simulink model "karol_kanoniczny"  (R2021b)
settings: Solver=VariableStepAuto  StartTime=0.0  StopTime=10.0  RelTol=1e-3
settings Model: Creator=radek  LastModifiedBy=radek

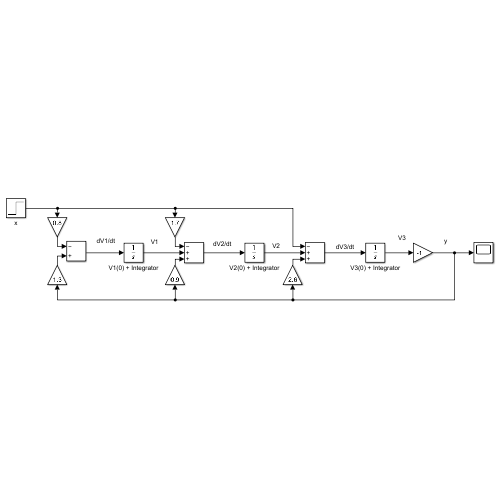
[thumbnail: Simulink's stored preview of the top-level diagram]
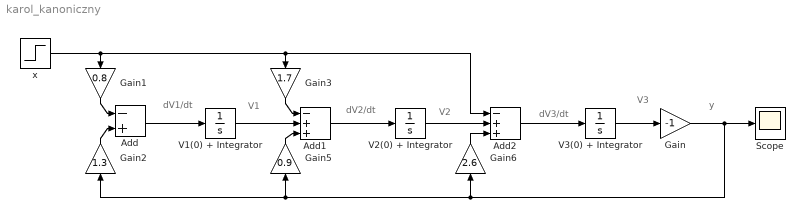
== system karol_kanoniczny ==
  note: y
  note: V3
  note: dV3/dt
  note: V2
  note: dV2/dt
  note: V1
  note: dV1/dt
  Add : Sum  Inputs=-+
  Add1 : Sum  Inputs=-++
  Add2 : Sum  Inputs=-++
  Gain : Gain  Gain=-1
  Gain1 : Gain  Gain=0.8
  Gain2 : Gain  Gain=1.3
  Gain3 : Gain  Gain=1.7
  Gain5 : Gain  Gain=0.9
  Gain6 : Gain  Gain=2.6
  Scope : Scope
  V1(0) + Integrator : Integrator
  V2(0) + Integrator : Integrator
  V3(0) + Integrator : Integrator
  x : Step  SampleTime=0
  wires:
  Gain1/1 -> Add/1
  Gain2/1 -> Add/2
  Add/1 -> V1(0) + Integrator/1
  V1(0) + Integrator/1 -> Add1/2
  Gain3/1 -> Add1/1
  Add1/1 -> V2(0) + Integrator/1
  V2(0) + Integrator/1 -> Add2/2
  x/1 -> Add2/1, Gain3/1, Gain1/1
  Add2/1 -> V3(0) + Integrator/1
  V3(0) + Integrator/1 -> Gain/1
  Gain/1 -> Gain6/1, Gain2/1, Gain5/1, Scope/1
  Gain5/1 -> Add1/3
  Gain6/1 -> Add2/3
